simulink model "dec_dly_comp"  (R2023b)
settings: Solver=VariableStepDiscrete  StartTime=0.0  StopTime=DDC_LINEUP_param.endTime  RelTol=1e-3  EnableMultiTasking=on
PreLoadFcn:
  | % Run the setup script when the model is opened
  | setup_dec_dly_comp;
InitFcn:
  | % Run the setup script again just before the
  | % model is run, so that any updates made
  | % after opening are applied.
  | 
  | setup_dec_dly_comp;
StopFcn:
  | dec_dly_comp_output_analysis;
undefined symbols (not defined in the file or in its folder): AdvDSPBChannelOutDisplay, AdvDSPBDMemDisplay, DDC_LINEUP_param, dpoly, dspba_ChannelInVis, dspba_ChannelOutVis, dspba_internal_get_channel_ports, evalAionMaskParam, latency, primtype, UseDontCare, value
libraries: DSPBAPrim x52, DSPBAModelBus x14, DSPBABase x10, simulink x9, DSPBAFilters x2
(part 2 of 2)

== system dec_dly_comp/DUT/DUT/Antenna_Gain Delay Compensation/Delay Compensation/TraceAntennaData1 ==
  DataIn : Inport
  ChIn : Inport  Port=2
  Enable : EnablePort
  DucAntDataOut : ToWorkspace  VariableName=AntGain_dOut  SampleTime=-1
  DucAntDataOut1 : ToWorkspace  VariableName=AntGain_cOut  SampleTime=-1
  wires:
  ChIn/1 -> DucAntDataOut1/1
  DataIn/1 -> DucAntDataOut/1

== system dec_dly_comp/DUT/DUT/Antenna_Gain Delay Compensation/Delay Compensation/TraceAntennaData4 ==
  DataIn : Inport
  ChIn : Inport  Port=2
  Enable : EnablePort
  DucAntDataOut : ToWorkspace  VariableName=AntGain_dIn  SampleTime=-1
  DucAntDataOut1 : ToWorkspace  VariableName=AntGain_cIn  SampleTime=-1
  wires:
  DataIn/1 -> DucAntDataOut/1
  ChIn/1 -> DucAntDataOut1/1
